simulink subsystem "kalman_filter"  (R2024b)
settings: Solver=VariableStepAuto  StartTime=0.0  StopTime=10.0  RelTol=1e-3
undefined symbols (not defined in the file or in its folder): airdata, Discrete, GROUND_LEVEL, input_rate, kalm_ffwd, kalm_initial, kalm_input, kalm_meas_cov, kalm_output, kalm_process_cov, kalm_state, Time, use_custom_atm
libraries: simulink x1, ctrlSharedLib x1
settings Model: Creator=yevge  LastModifiedBy=Aiden Gaydos

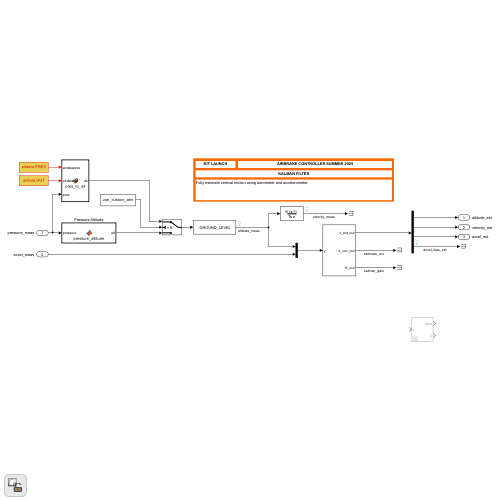
[thumbnail: Simulink's stored preview of the top-level diagram]
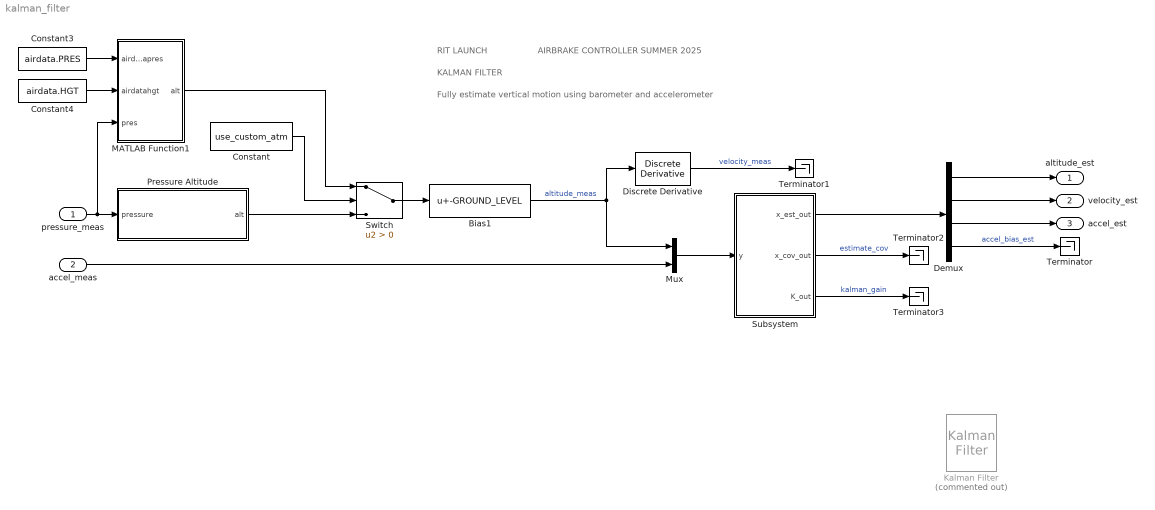
== system kalman_filter ==
  note: KALMAN FILTER
  note: Fully estimate vertical motion using barometer and accelerometer
  note: RIT LAUNCH
  note: AIRBRAKE CONTROLLER SUMMER 2025
  pressure_meas : Inport  PortDimensions=1
  accel_meas : Inport  Port=2  PortDimensions=1
  Bias1 : Bias  Bias=-GROUND_LEVEL  SaturateOnIntegerOverflow=off
  Constant : Constant  Value=use_custom_atm
  Constant3 : Constant  Value=airdata.PRES
  Constant4 : Constant  Value=airdata.HGT
  Demux : Demux
  Discrete Derivative : simulink/Discrete/Discrete Derivative  gainval=1  ICPrevScaledInput=0.0  OutMin=[]  OutMax=[]  OutDataType=fixdt(1, 16)  OutScaling=2^-10  DoSatur=off
  Kalman Filter : ctrlSharedLib/Kalman Filter  Commented=on  TimeDomain=Discrete-Time  UseCurrentEstimator=on  ModelSource=Individual A, B, C, D matrices  ModelSourceVariable=ss(0.95,1,1,0,1)  A=kalm_state  B=kalm_input  C=kalm_output  D=kalm_ffwd  NumberOfStates=1  NumberOfInputs=1  NumberOfOutputs=1  InitialEstimateSource=Dialog  X0=kalm_initial  P0=10  UseK=off  UseGH=off  NumberOfProcessNoiseInputs=1  G=1  TimeInvariantG=on  H=0  TimeInvariantH=on  Q=kalm_process_cov  TimeInvariantQ=on  R=kalm_meas_cov  TimeInvariantR=on  N=0  TimeInvariantN=on  AddInputPort=off  AddEnablePort=off  OutputEstimatedY=off  OutputP=on  Ts=1/input_rate
  MATLAB Function1 : MATLAB Function  TreatAsAtomicUnit=on
  Mux : Mux  Inputs=2
  Pressure Altitude : MATLAB Function  TreatAsAtomicUnit=on
  Subsystem : Subsystem  mask{kalm_sample_rate=input_rate, kalm_state_matrix=kalm_state, kalm_state_cov=kalm_process_cov, kalm_measure_matrix=kalm_output, kalm_measure_cov=kalm_meas_cov, kalm_initial_state=kalm_initial, kalm_initial_cov=eye(length(kalm_initial))}
      mask prompts: kalm_sample_rate "Sample rate"; kalm_state_matrix "State matrix"; kalm_state_cov "State covariance"; kalm_measure_matrix "Measurement matrix"; kalm_measure_cov "Measurement covariance"; kalm_initial_state "Initial state"; kalm_initial_cov "Initial estimate covariance"
  Switch : Switch  Criteria=u2 > Threshold  SaturateOnIntegerOverflow=off  InputSameDT=off
  Terminator{,1..3} (4 alike) : Terminator
  altitude_est : Outport  PortDimensions=1
  velocity_est : Outport  Port=2  PortDimensions=1
  accel_est : Outport  Port=3  PortDimensions=1
  wires:
  Demux/2 -> velocity_est/1
  Demux/1 -> altitude_est/1
  accel_meas/1 -> Mux/2
  Demux/3 -> accel_est/1
  Mux/1 -> Subsystem/1(y)
  Demux/4 -> Terminator/1  "accel_bias_est"
  pressure_meas/1 -> Pressure Altitude/1(pressure), MATLAB Function1/3(pres)
  Bias1/1 -> Discrete Derivative/1, Mux/1  "altitude_meas"
  Subsystem/1(x_est_out) -> Demux/1
  Discrete Derivative/1 -> Terminator1/1  "velocity_meas"
  Subsystem/2(x_cov_out) -> Terminator2/1  "estimate_cov"
  Subsystem/3(K_out) -> Terminator3/1  "kalman_gain"
  Constant3/1 -> MATLAB Function1/1(airdatapres)
  Constant4/1 -> MATLAB Function1/2(airdatahgt)
  Switch/1 -> Bias1/1
  Constant/1 -> Switch/2
  MATLAB Function1/1(alt) -> Switch/1
  Pressure Altitude/1(alt) -> Switch/3

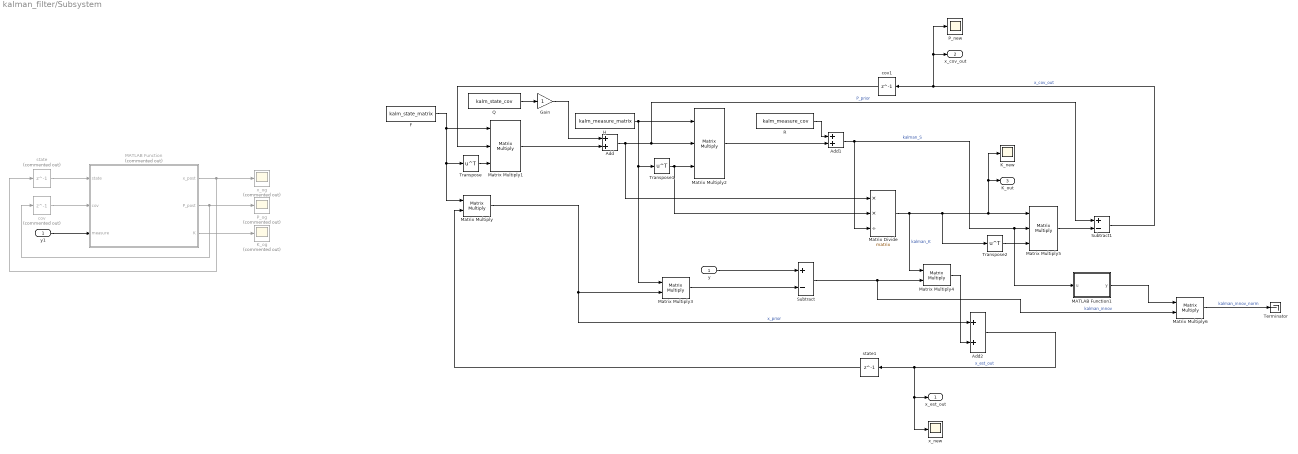
== system kalman_filter/Subsystem ==
  y : Inport  SampleTime=1/kalm_sample_rate
  Add : Sum
  Add1 : Sum
  Add2 : Sum
  F : Constant  Value=kalm_state_matrix
  Gain : Gain
  H : Constant  Value=kalm_measure_matrix
  K_new : Scope
  K_og : Scope  Commented=on
  MATLAB Function : MATLAB Function  Commented=on  TreatAsAtomicUnit=on
  MATLAB Function1 : MATLAB Function  TreatAsAtomicUnit=on
  Matrix Divide : Product  Inputs=**/  Multiplication=Matrix(*)
  Matrix Multiply{,3..4,6} (4 alike) : Product  Multiplication=Matrix(*)
  Matrix Multiply1 : Product  Inputs=3  Multiplication=Matrix(*)
  Matrix Multiply2 : Product  Inputs=3  Multiplication=Matrix(*)
  Matrix Multiply5 : Product  Inputs=3  Multiplication=Matrix(*)
  P_new : Scope
  P_og : Scope  Commented=on
  Q : Constant  Value=kalm_state_cov
  R : Constant  Value=kalm_measure_cov
  Subtract : Sum  Inputs=+-
  Subtract1 : Sum  Inputs=+-
  Terminator : Terminator
  Transpose : Math  Operator=transpose
  Transpose1 : Math  Operator=transpose
  Transpose2 : Math  Operator=transpose
  cov : Delay  Commented=on  DelayLength=1  InitialCondition=kalm_initial_cov  SampleTime=1/kalm_sample_rate
  cov1 : Delay  DelayLength=1  InitialCondition=kalm_initial_cov  SampleTime=1/kalm_sample_rate
  state : Delay  Commented=on  DelayLength=1  InitialCondition=kalm_initial_state  SampleTime=1/kalm_sample_rate
  state1 : Delay  DelayLength=1  InitialCondition=kalm_initial_state  SampleTime=1/kalm_sample_rate
  x_new : Scope
  x_og : Scope  Commented=on
  y1 : InportShadow  SampleTime=1/kalm_sample_rate
  x_est_out : Outport  SampleTime=1/kalm_sample_rate
  x_cov_out : Outport  Port=2  SampleTime=1/kalm_sample_rate
  K_out : Outport  Port=3  SampleTime=1/kalm_sample_rate
  wires:
  MATLAB Function/3(K) -> K_og/1
  y1/1 -> MATLAB Function/3(measure)
  y/1 -> Subtract/1
  state1/1 -> Matrix Multiply/2
  Matrix Multiply2/1 -> Add1/2
  Add/1 -> Matrix Divide/1, Subtract1/1, Matrix Multiply2/2  "P_prior"
  Transpose/1 -> Matrix Multiply1/3
  Matrix Multiply4/1 -> Add2/2
  H/1 -> Matrix Multiply2/1, Matrix Multiply3/1, Transpose1/1
  Subtract1/1 -> cov1/1, x_cov_out/1, P_new/1  "x_cov_out"
  Matrix Multiply1/1 -> Add/2
  MATLAB Function1/1(y) -> Matrix Multiply6/1
  Add1/1 -> MATLAB Function1/1(u), Matrix Multiply5/2, Matrix Divide/3  "kalman_S"
  Subtract/1 -> Matrix Multiply6/2, Matrix Multiply4/2  "kalman_innov"
  Matrix Multiply5/1 -> Subtract1/2
  R/1 -> Add1/1
  Matrix Multiply/1 -> Add2/1, Matrix Multiply3/2  "x_prior"
  Matrix Multiply3/1 -> Subtract/2
  Matrix Divide/1 -> Matrix Multiply4/1, Transpose2/1, K_out/1, K_new/1, Matrix Multiply5/1  "kalman_K"
  F/1 -> Matrix Multiply/1, Transpose/1, Matrix Multiply1/1
  Transpose2/1 -> Matrix Multiply5/3
  Matrix Multiply6/1 -> Terminator/1  "kalman_innov_norm"
  Add2/1 -> state1/1, x_est_out/1, x_new/1  "x_est_out"
  Transpose1/1 -> Matrix Divide/2, Matrix Multiply2/3
  cov1/1 -> Matrix Multiply1/2
  Q/1 -> Gain/1
  Gain/1 -> Add/1
  state/1 -> MATLAB Function/1(state)
  MATLAB Function/2(P_post) -> P_og/1, cov/1
  cov/1 -> MATLAB Function/2(cov)
  MATLAB Function/1(x_post) -> state/1, x_og/1

== matlab function kalman_filter/Pressure Altitude ==
  data: pressure input; alt output
function alt = pressure_altitude(pressure)
    alt = (1 - (pressure ./ 101325).^(0.190284)) .* 145366.45 * 0.3048;
end

== matlab function kalman_filter/Subsystem/MATLAB Function ==
  data: state input size=size(kalm_state_matrix, 1); cov input size=size(kalm_state_matrix); measure input size=size(kalm_measure_matrix,1); x_post output size=size(kalm_state_matrix, 1); P_post output size=size(kalm_state_matrix); K output size=[size(kalm_state_matrix,1), size(kalm_measure_matrix, 1)]; kalm_state_matrix parameter; kalm_state_cov parameter size=size(kalm_state_matrix); kalm_measure_matrix parameter; kalm_measure_cov parameter size=[size(kalm_measure_matrix, 1), size(kalm_measure_matrix, 1)]
function [x_post, P_post, K] = kalman_update(state, cov, measure, ...
    kalm_state_matrix, kalm_state_cov, ...
    kalm_measure_matrix, kalm_measure_cov)

% using nomenclature from https://en.wikipedia.org/wiki/Kalman_filter
    % Rename variables
    x = state;
    P = cov;
    z = measure;

    F = kalm_state_matrix;
    Q = kalm_state_cov;
    H = kalm_measure_matrix;
    R = kalm_measure_cov;
    
    % Calculate priors
    x_prior = F * x;
    P_prior = F * P * (F.') + Q;

    S = H * P_prior * (H.') + R;
    K = P_prior * (H.') / S;

    % Calculate outputs
    K_comp = eye(length(x)) - K * H; % complement of Kalman gain
    x_post = K_comp * x_prior + K * z;
    P_post = K_comp * P_prior;
end

== matlab function kalman_filter/MATLAB Function1 ==
  data: airdatapres input; airdatahgt input; pres input; alt output
function alt = pres_to_alt(airdatapres,airdatahgt,pres)
    alt = double(interp1(airdatapres,airdatahgt,pres,"linear","extrap"));
end

== matlab function kalman_filter/Subsystem/MATLAB Function1 ==
  data: u input; y output
function y = fcn(u)

y = inv(sqrtm(u));
